simulink model "nolinear_controller_compare"  (R2023a)
settings: Solver=VariableStepAuto  StartTime=0.0  StopTime=50  RelTol=1e-3
settings Model: Creator=belov  LastModifiedBy=belov

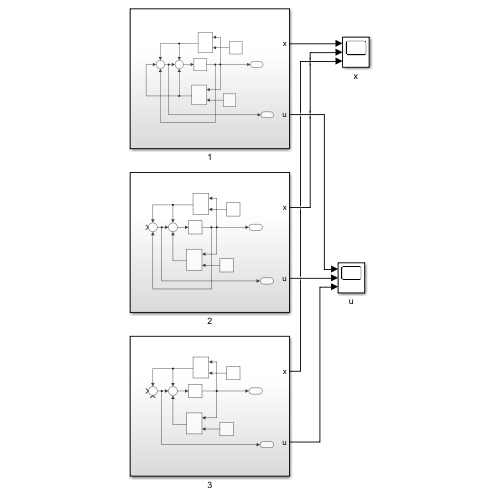
[thumbnail: Simulink's stored preview of the top-level diagram]
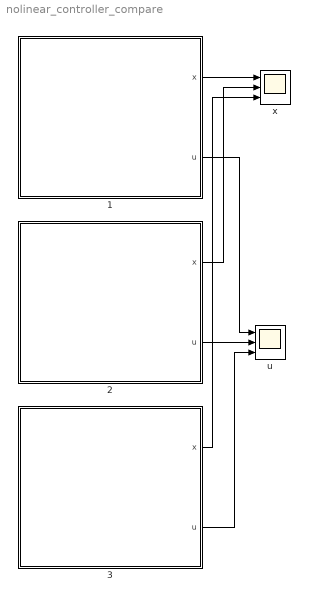
== system nolinear_controller_compare ==
  1 : Subsystem
  2 : Subsystem
  3 : Subsystem
  u : Scope  NumInputPorts=3
  x : Scope  NumInputPorts=3
  wires:
  2/2(u) -> u/2
  1/2(u) -> u/1
  3/2(u) -> u/3
  1/1(x) -> x/1
  2/1(x) -> x/2
  3/1(x) -> x/3

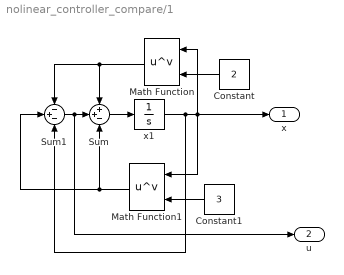
== system nolinear_controller_compare/1 ==
  Constant : Constant  Value=2
  Constant1 : Constant  Value=3
  Math Function : Math  Operator=pow
  Math Function1 : Math  Operator=pow
  Sum : Sum  Inputs=++-
  Sum1 : Sum  Inputs=-+-
  x1 : Integrator  InitialCondition=1
  x : Outport
  u : Outport  Port=2
  wires:
  Math Function/1 -> Sum/1, Sum1/1
  x1/1 -> Sum1/3, x/1, Math Function1/1, Math Function/1
  Constant1/1 -> Math Function1/2
  Sum/1 -> x1/1
  Math Function1/1 -> Sum1/2, Sum/3
  Constant/1 -> Math Function/2
  Sum1/1 -> u/1, Sum/2

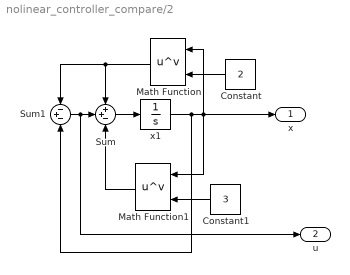
== system nolinear_controller_compare/2 ==
  Constant : Constant  Value=2
  Constant1 : Constant  Value=3
  Math Function : Math  Operator=pow
  Math Function1 : Math  Operator=pow
  Sum : Sum  Inputs=++-
  Sum1 : Sum  Inputs=-+-
  x1 : Integrator  InitialCondition=1
  x : Outport
  u : Outport  Port=2
  wires:
  Sum1/1 -> Sum/2, u/1
  Constant/1 -> Math Function/2
  Math Function1/1 -> Sum/3
  Sum/1 -> x1/1
  Constant1/1 -> Math Function1/2
  x1/1 -> Math Function/1, Math Function1/1, x/1, Sum1/3
  Math Function/1 -> Sum1/1, Sum/1

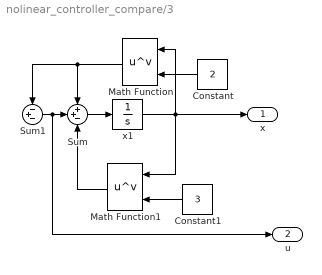
== system nolinear_controller_compare/3 ==
  Constant : Constant  Value=2
  Constant1 : Constant  Value=3
  Math Function : Math  Operator=pow
  Math Function1 : Math  Operator=pow
  Sum : Sum  Inputs=++-
  Sum1 : Sum  Inputs=-+-
  x1 : Integrator  InitialCondition=1
  x : Outport
  u : Outport  Port=2
  wires:
  Math Function/1 -> Sum/1, Sum1/1
  x1/1 -> x/1, Math Function1/1, Math Function/1
  Constant1/1 -> Math Function1/2
  Sum/1 -> x1/1
  Math Function1/1 -> Sum/3
  Constant/1 -> Math Function/2
  Sum1/1 -> u/1, Sum/2
